simulink model "teleoperation"  (Simulink 9.3)
settings: Solver=ode4  StartTime=0.0  StopTime=2  FixedStep=0.0001  RelTol=1e-3
model workspace: external: MATLAB Code (data not in the file)
libraries: simulink x3
settings Model: Creator=z-lu  LastModifiedBy=luzhe
settings DataIOCC: SaveFormat=Dataset  SignalLoggingSaveFormat=Dataset  ReturnWorkspaceOutputs=on
settings DebuggingCC: UnderspecifiedInitializationDetection=Simplified  MergeDetectMultiDrivingBlocksExec=error  FcnCallInpInsideContextMsg=error  SFUnexpectedBacktrackingDiag=error  SFNoUnconditionalDefaultTransitionDiag=error
settings HardwareCC: ProdBitPerPointer=64  ProdLargestAtomicFloat=Float  ProdIntDivRoundTo=Zero  ProdEndianess=LittleEndian  ProdHWDeviceType=Specified
settings ModelReferenceCC: PropagateSignalLabelsOutOfModel=on
settings SFSimCC: SimUseLocalCustomCode=on
settings RTWCC: RTWUseLocalCustomCode=on
settings GRTTargetCC: TargetLangStandard=C99 (ISO)  CombineOutputUpdateFcns=on  GRTInterface=off
settings ConfigComp: CovMetricSettings=dwe  CovHtmlReporting=off  CovSaveCumulativeToWorkspaceVar=off  CovSaveSingleToWorkspaceVar=off  CovExternalEMLEnable=on

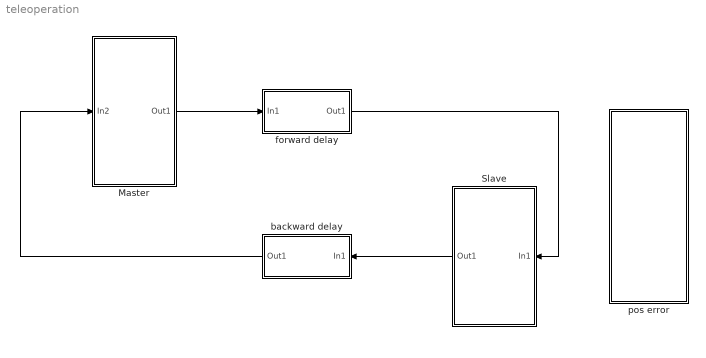
== system teleoperation ==
  "Master " : Subsystem
  Slave : Subsystem
  backward delay : Subsystem
  forward delay : Subsystem
  pos error : Subsystem
  wires:
  forward delay/1(Out1) -> Slave/1(In1)
  Slave/1(Out1) -> backward delay/1(In1)
  backward delay/1(Out1) -> "Master "/1(In2)
  "Master "/1(Out1) -> forward delay/1(In1)

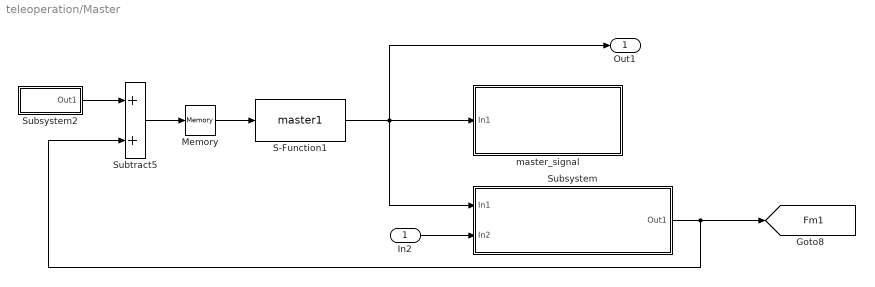
== system teleoperation/Master  ==
  In2 : Inport
  Memory : Memory  InheritSampleTime=on
  S-Function1 : S-Function  FunctionName=master1  SFunctionDeploymentMode=off  EnableBusSupport=off
  Subsystem : Subsystem
  Subsystem2 : Subsystem
  Subtract5 : Sum
  master_signal : Subsystem
  Out1 : Outport
  tag scope: Fm1=global
  wires:
  Memory/1 -> S-Function1/1
  Subsystem/1(Out1) -> Subtract5/2, [Fm1]
  S-Function1/1 -> Out1/1, master_signal/1(In1), Subsystem/1(In1)
  Subtract5/1 -> Memory/1
  In2/1 -> Subsystem/2(In2)
  Subsystem2/1(Out1) -> Subtract5/1

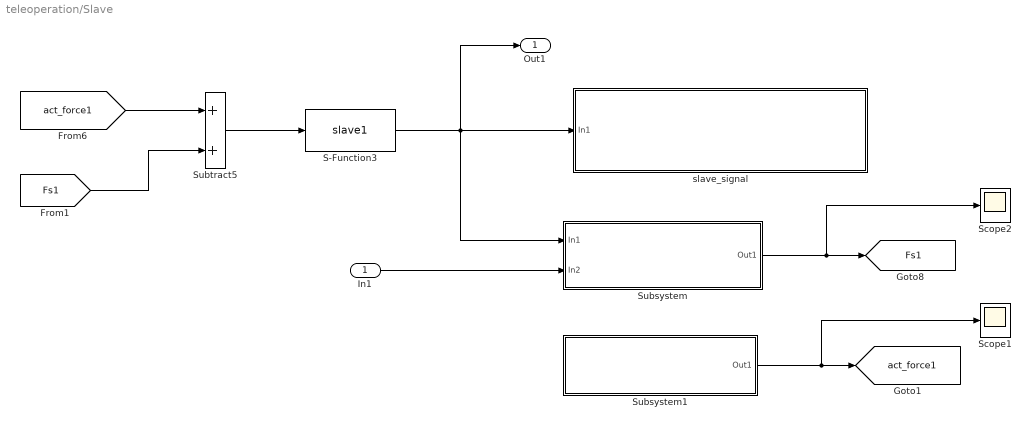
== system teleoperation/Slave ==
  In1 : Inport
  S-Function3 : S-Function  FunctionName=slave1  SFunctionDeploymentMode=off  EnableBusSupport=off
  Scope1 : Scope
  Scope2 : Scope
  Subsystem : Subsystem
  Subsystem1 : Subsystem
  Subtract5 : Sum
  slave_signal : Subsystem
  Out1 : Outport
  tag scope: Fs1=global, act_force1=global
  wires:
  Subsystem/1(Out1) -> Scope2/1, [Fs1]
  Subtract5/1 -> S-Function3/1
  In1/1 -> Subsystem/2(In2)
  [Fs1] -> Subtract5/2
  Subsystem1/1(Out1) -> Scope1/1, [act_force1]
  S-Function3/1 -> Out1/1, Subsystem/1(In1), slave_signal/1(In1)
  [act_force1] -> Subtract5/1

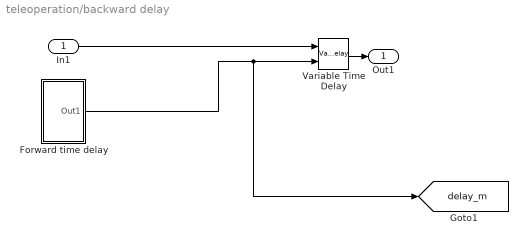
== system teleoperation/backward delay ==
  In1 : Inport
  Forward time delay : Subsystem
  Variable Time Delay : VariableTransportDelay  MaximumDelay=10
  Out1 : Outport
  tag scope: delay_m=global
  wires:
  Variable Time Delay/1 -> Out1/1
  In1/1 -> Variable Time Delay/1
  Forward time delay/1(Out1) -> [delay_m], Variable Time Delay/2

== system teleoperation/forward delay ==
  In1 : Inport
  Forward time delay : Subsystem
  Variable Time Delay : VariableTransportDelay  MaximumDelay=10
  Out1 : Outport
  tag scope: fmq1=global
  wires:
  In1/1 -> [fmq1], Variable Time Delay/1
  Variable Time Delay/1 -> Out1/1
  Forward time delay/1(Out1) -> Variable Time Delay/2

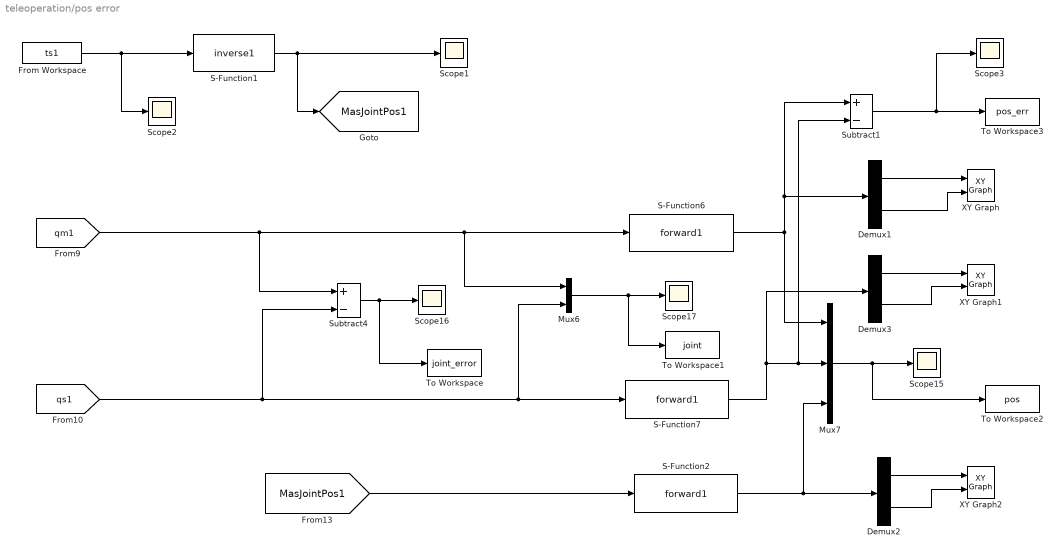
== system teleoperation/pos error ==
  Demux1 : Demux  Outputs=2
  Demux2 : Demux  Outputs=2
  Demux3 : Demux  Outputs=2
  From Workspace : FromWorkspace  VariableName=ts1  SampleTime=0
  Mux6 : Mux  Inputs=2
  Mux7 : Mux  Inputs=3
  S-Function1 : S-Function  FunctionName=inverse1  SFunctionDeploymentMode=off  EnableBusSupport=off
  S-Function2 : S-Function  FunctionName=forward1  SFunctionDeploymentMode=off  EnableBusSupport=off
  S-Function6 : S-Function  FunctionName=forward1  SFunctionDeploymentMode=off  EnableBusSupport=off
  S-Function7 : S-Function  FunctionName=forward1  SFunctionDeploymentMode=off  EnableBusSupport=off
  Scope{1..3,15..17} (6 alike) : Scope
  Subtract1 : Sum  Inputs=+-
  Subtract4 : Sum  Inputs=+-
  To Workspace : ToWorkspace  VariableName=joint_error  SaveFormat=Timeseries  SampleTime=-1
  To Workspace1 : ToWorkspace  VariableName=joint  SaveFormat=Timeseries  SampleTime=-1
  To Workspace2 : ToWorkspace  VariableName=pos  SaveFormat=Timeseries  SampleTime=-1
  To Workspace3 : ToWorkspace  VariableName=pos_err  SaveFormat=Timeseries  SampleTime=-1
  XY Graph : simulink/Sinks/XY Graph  xmin=-1  xmax=1  ymin=-1  ymax=1  st=-1
  XY Graph1 : simulink/Sinks/XY Graph  xmin=-1  xmax=1  ymin=-1  ymax=1  st=-1
  XY Graph2 : simulink/Sinks/XY Graph  xmin=-1  xmax=1  ymin=-1  ymax=1  st=-1
  tag scope: MasJointPos1=global
  wires:
  Mux6/1 -> To Workspace1/1, Scope17/1
  S-Function6/1 -> Demux1/1, Subtract1/1, Mux7/1
  [qs1] -> Subtract4/2, S-Function7/1, Mux6/2
  Mux7/1 -> To Workspace2/1, Scope15/1
  Subtract4/1 -> To Workspace/1, Scope16/1
  S-Function1/1 -> Scope1/1, [MasJointPos1]
  S-Function2/1 -> Mux7/3, Demux2/1
  [qm1] -> Subtract4/1, Mux6/1, S-Function6/1
  Subtract1/1 -> Scope3/1, To Workspace3/1
  From Workspace/1 -> Scope2/1, S-Function1/1
  [MasJointPos1] -> S-Function2/1
  Demux1/1 -> XY Graph/1
  Demux1/2 -> XY Graph/2
  Demux2/1 -> XY Graph2/1
  Demux2/2 -> XY Graph2/2
  Demux3/2 -> XY Graph1/2
  Demux3/1 -> XY Graph1/1
  S-Function7/1 -> Demux3/1, Subtract1/2, Mux7/2

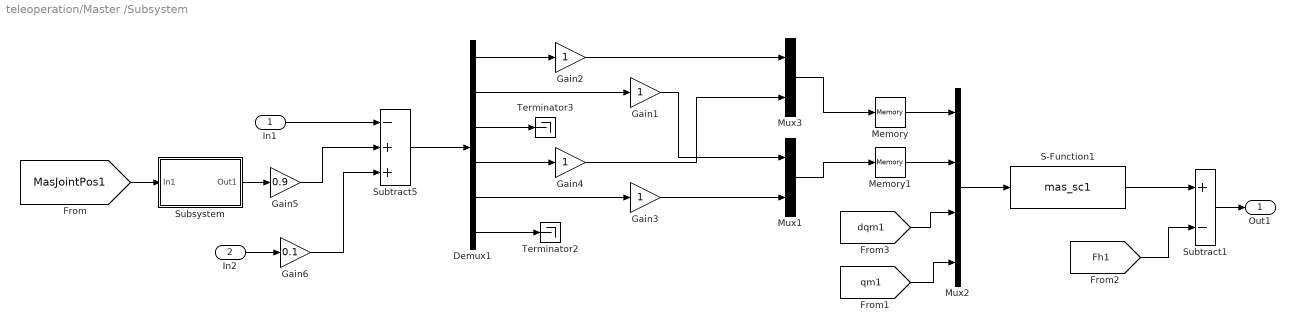
== system teleoperation/Master /Subsystem ==
  In1 : Inport
  In2 : Inport  Port=2
  Demux1 : Demux  Outputs=6
  Gain{1..4} (4 alike) : Gain
  Gain5 : Gain  Gain=0.9
  Gain6 : Gain  Gain=0.1
  Memory : Memory
  Memory1 : Memory
  Mux1 : Mux  Inputs=2
  Mux2 : Mux
  Mux3 : Mux  Inputs=2
  S-Function1 : S-Function  FunctionName=mas_sc1  SFunctionDeploymentMode=off  EnableBusSupport=off
  Subsystem : Subsystem
  Subtract1 : Sum  Inputs=+-
  Subtract5 : Sum  Inputs=-++
  Terminator2 : Terminator
  Terminator3 : Terminator
  Out1 : Outport
  wires:
  In1/1 -> Subtract5/1
  Subtract5/1 -> Demux1/1
  Demux1/6 -> Terminator2/1
  Demux1/3 -> Terminator3/1
  S-Function1/1 -> Subtract1/1
  Mux2/1 -> S-Function1/1
  Demux1/1 -> Gain2/1
  Demux1/4 -> Gain4/1
  Demux1/2 -> Gain1/1
  Demux1/5 -> Gain3/1
  Mux3/1 -> Memory/1
  Gain2/1 -> Mux3/1
  Gain4/1 -> Mux3/2
  Gain1/1 -> Mux1/1
  Gain3/1 -> Mux1/2
  Mux1/1 -> Memory1/1
  [dqm1] -> Mux2/3
  Memory/1 -> Mux2/1
  Memory1/1 -> Mux2/2
  [qm1] -> Mux2/4
  [MasJointPos1] -> Subsystem/1(In1)
  Subsystem/1(Out1) -> Gain5/1
  Gain5/1 -> Subtract5/2
  In2/1 -> Gain6/1
  Gain6/1 -> Subtract5/3
  Subtract1/1 -> Out1/1
  [Fh1] -> Subtract1/2

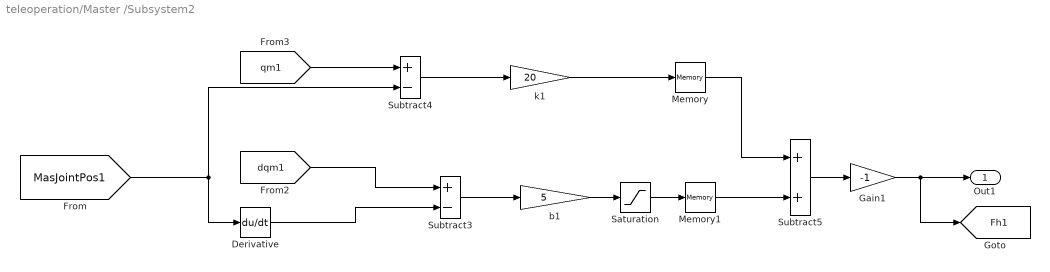
== system teleoperation/Master /Subsystem2 ==
  Derivative : Derivative
  Gain1 : Gain  Gain=-1
  Memory : Memory  InheritSampleTime=on
  Memory1 : Memory  InheritSampleTime=on
  Saturation : Saturate  UpperLimit=10  LowerLimit=-10
  Subtract3 : Sum  Inputs=+-
  Subtract4 : Sum  Inputs=+-
  Subtract5 : Sum
  b1 : Gain  Gain=5
  k1 : Gain  Gain=20
  Out1 : Outport
  tag scope: Fh1=global
  wires:
  Memory1/1 -> Subtract5/2
  [MasJointPos1] -> Subtract4/2, Derivative/1
  Memory/1 -> Subtract5/1
  Subtract5/1 -> Gain1/1
  k1/1 -> Memory/1
  [dqm1] -> Subtract3/1
  Gain1/1 -> [Fh1], Out1/1
  Derivative/1 -> Subtract3/2
  [qm1] -> Subtract4/1
  Subtract4/1 -> k1/1
  Subtract3/1 -> b1/1
  b1/1 -> Saturation/1
  Saturation/1 -> Memory1/1

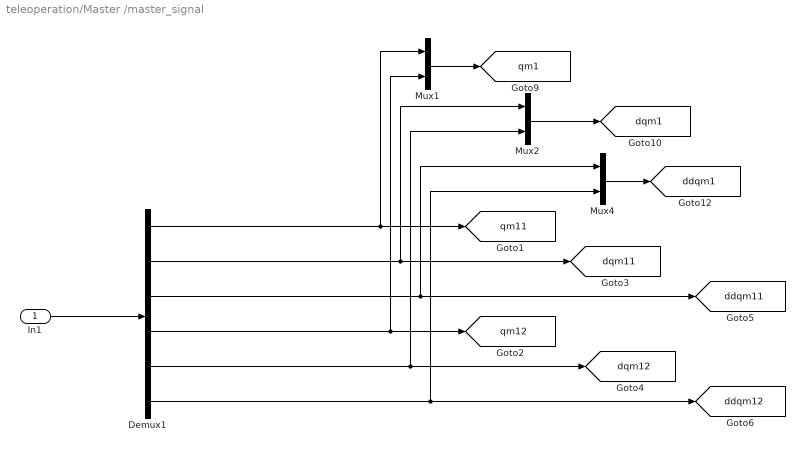
== system teleoperation/Master /master_signal ==
  In1 : Inport
  Demux1 : Demux  Outputs=6
  Mux1 : Mux  Inputs=2
  Mux2 : Mux  Inputs=2
  Mux4 : Mux  Inputs=2
  tag scope: ddqm11=global, ddqm12=global, ddqm1=global, dqm11=global, dqm12=global, dqm1=global, qm11=global, qm12=global, qm1=global
  wires:
  Demux1/2 -> [dqm11], Mux2/1
  Demux1/5 -> [dqm12], Mux2/2
  Demux1/6 -> [ddqm12], Mux4/2
  Demux1/4 -> [qm12], Mux1/2
  Mux1/1 -> [qm1]
  In1/1 -> Demux1/1
  Mux2/1 -> [dqm1]
  Demux1/1 -> [qm11], Mux1/1
  Demux1/3 -> [ddqm11], Mux4/1
  Mux4/1 -> [ddqm1]

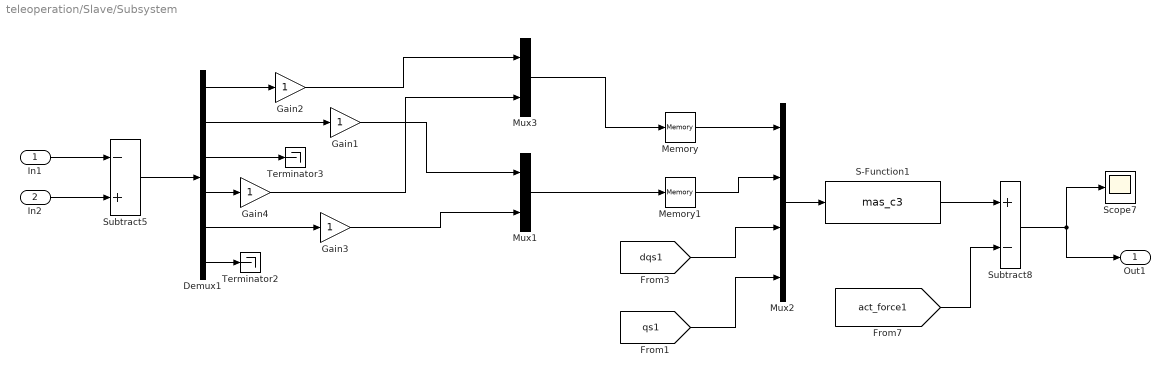
== system teleoperation/Slave/Subsystem ==
  In1 : Inport
  In2 : Inport  Port=2
  Demux1 : Demux  Outputs=6
  Gain{1..4} (4 alike) : Gain
  Memory : Memory
  Memory1 : Memory
  Mux1 : Mux  Inputs=2
  Mux2 : Mux
  Mux3 : Mux  Inputs=2
  S-Function1 : S-Function  FunctionName=mas_c3  SFunctionDeploymentMode=off  EnableBusSupport=off
  Scope7 : Scope
  Subtract5 : Sum  Inputs=-+
  Subtract8 : Sum  Inputs=+-
  Terminator2 : Terminator
  Terminator3 : Terminator
  Out1 : Outport
  wires:
  In1/1 -> Subtract5/1
  In2/1 -> Subtract5/2
  Subtract5/1 -> Demux1/1
  Demux1/6 -> Terminator2/1
  Demux1/3 -> Terminator3/1
  Subtract8/1 -> Scope7/1, Out1/1
  Mux2/1 -> S-Function1/1
  Demux1/1 -> Gain2/1
  Demux1/4 -> Gain4/1
  Demux1/2 -> Gain1/1
  Demux1/5 -> Gain3/1
  Memory/1 -> Mux2/1
  S-Function1/1 -> Subtract8/1
  Memory1/1 -> Mux2/2
  Gain2/1 -> Mux3/1
  Mux3/1 -> Memory/1
  Gain1/1 -> Mux1/1
  Mux1/1 -> Memory1/1
  Gain3/1 -> Mux1/2
  Gain4/1 -> Mux3/2
  [dqs1] -> Mux2/3
  [qs1] -> Mux2/4
  [act_force1] -> Subtract8/2

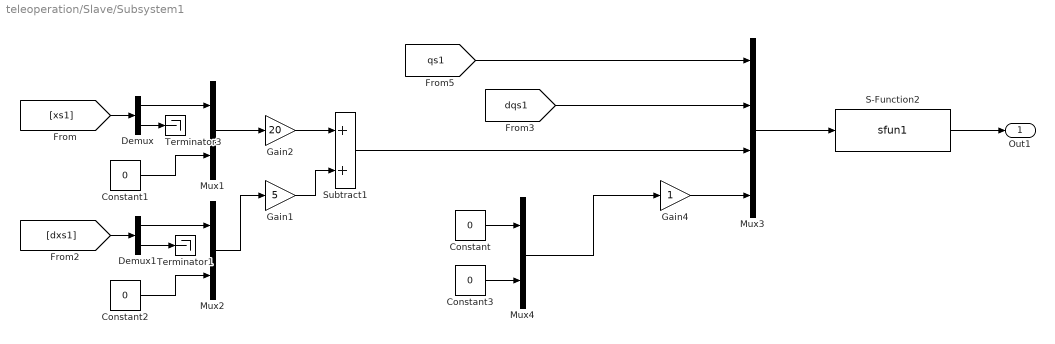
== system teleoperation/Slave/Subsystem1 ==
  Constant{,1..3} (4 alike) : Constant  Value=0
  Demux : Demux  Outputs=2
  Demux1 : Demux  Outputs=2
  Gain1 : Gain  Gain=5
  Gain2 : Gain  Gain=20
  Gain4 : Gain
  Mux1 : Mux  Inputs=2
  Mux2 : Mux  Inputs=2
  Mux3 : Mux
  Mux4 : Mux  Inputs=2
  S-Function2 : S-Function  FunctionName=sfun1  SFunctionDeploymentMode=off  EnableBusSupport=off
  Subtract1 : Sum
  Terminator1 : Terminator
  Terminator3 : Terminator
  Out1 : Outport
  wires:
  Demux/2 -> Terminator3/1
  Demux/1 -> Mux1/1
  [dxs1] -> Demux1/1
  [xs1] -> Demux/1
  Demux1/1 -> Mux2/1
  Demux1/2 -> Terminator1/1
  Constant1/1 -> Mux1/2
  Gain1/1 -> Subtract1/2
  Mux2/1 -> Gain1/1
  Mux1/1 -> Gain2/1
  Gain2/1 -> Subtract1/1
  Constant2/1 -> Mux2/2
  Mux3/1 -> S-Function2/1
  Constant/1 -> Mux4/1
  [qs1] -> Mux3/1
  [dqs1] -> Mux3/2
  Gain4/1 -> Mux3/4
  Constant3/1 -> Mux4/2
  S-Function2/1 -> Out1/1
  Mux4/1 -> Gain4/1
  Subtract1/1 -> Mux3/3

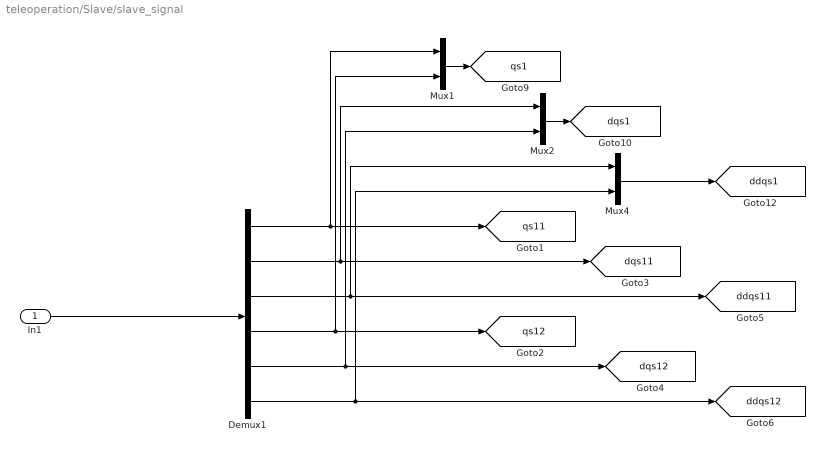
== system teleoperation/Slave/slave_signal ==
  In1 : Inport
  Demux1 : Demux  Outputs=6
  Mux1 : Mux  Inputs=2
  Mux2 : Mux  Inputs=2
  Mux4 : Mux  Inputs=2
  tag scope: ddqs11=global, ddqs12=global, ddqs1=global, dqs11=global, dqs12=global, dqs1=global, qs11=global, qs12=global, qs1=global
  wires:
  Demux1/5 -> [dqs12], Mux2/2
  In1/1 -> Demux1/1
  Demux1/6 -> [ddqs12], Mux4/2
  Mux4/1 -> [ddqs1]
  Mux2/1 -> [dqs1]
  Demux1/2 -> [dqs11], Mux2/1
  Demux1/4 -> [qs12], Mux1/2
  Demux1/1 -> [qs11], Mux1/1
  Demux1/3 -> [ddqs11], Mux4/1
  Mux1/1 -> [qs1]

== system teleoperation/backward delay/Forward time delay ==
  Constant4 : Constant  Value=0.001
  Out1 : Outport
  wires:
  Constant4/1 -> Out1/1

== system teleoperation/forward delay/Forward time delay ==
  Constant1 : Constant  Value=0.001
  Out1 : Outport
  wires:
  Constant1/1 -> Out1/1

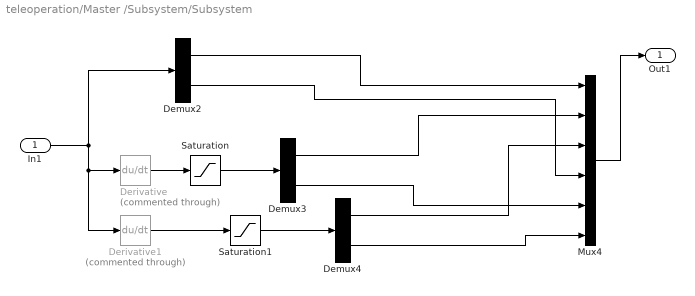
== system teleoperation/Master /Subsystem/Subsystem ==
  In1 : Inport
  Demux2 : Demux  Outputs=2
  Demux3 : Demux  Outputs=2
  Demux4 : Demux  Outputs=2
  Derivative : Derivative  Commented=through
  Derivative1 : Derivative  Commented=through
  Mux4 : Mux  Inputs=6
  Saturation : Saturate  UpperLimit=50  LowerLimit=-50
  Saturation1 : Saturate  UpperLimit=50  LowerLimit=-50
  Out1 : Outport
  wires:
  Demux3/1 -> Mux4/2
  Derivative1/1 -> Saturation1/1
  Demux2/1 -> Mux4/1
  In1/1 -> Demux2/1, Derivative1/1, Derivative/1
  Demux3/2 -> Mux4/5
  Mux4/1 -> Out1/1
  Demux4/1 -> Mux4/3
  Demux4/2 -> Mux4/6
  Derivative/1 -> Saturation/1
  Demux2/2 -> Mux4/4
  Saturation/1 -> Demux3/1
  Saturation1/1 -> Demux4/1
